simulink model "example"  (R2020b)
settings: Solver=ode45  StartTime=0.0  StopTime=10.0  RelTol=1e-3
InitFcn:
  | ac_testbed_setup
undefined symbols (not defined in the file): mpm, PD, QD, QG, VA, VM
libraries: SimMATPOWERbase x6, simulink x1
settings Model: Creator=hauswirth  LastModifiedBy=lukas
settings DataIOCC: SaveFormat=StructureWithTime  ReturnWorkspaceOutputs=off
settings OptimizationCC: LifeSpan=inf
settings DebuggingCC: SFExecutionAtInitializationDiag=none  ArithmeticOperatorsInVariantConditions=warning
settings HardwareCC: ProdBitPerSizeT=32  ProdBitPerPtrDiffT=32  ProdWordSize=32  ProdHWDeviceType=Specified
settings SFSimCC: CustomCodeUndefinedFunction=UseInterfaceOnly
settings CodeAppCC: StateflowObjectComments=on

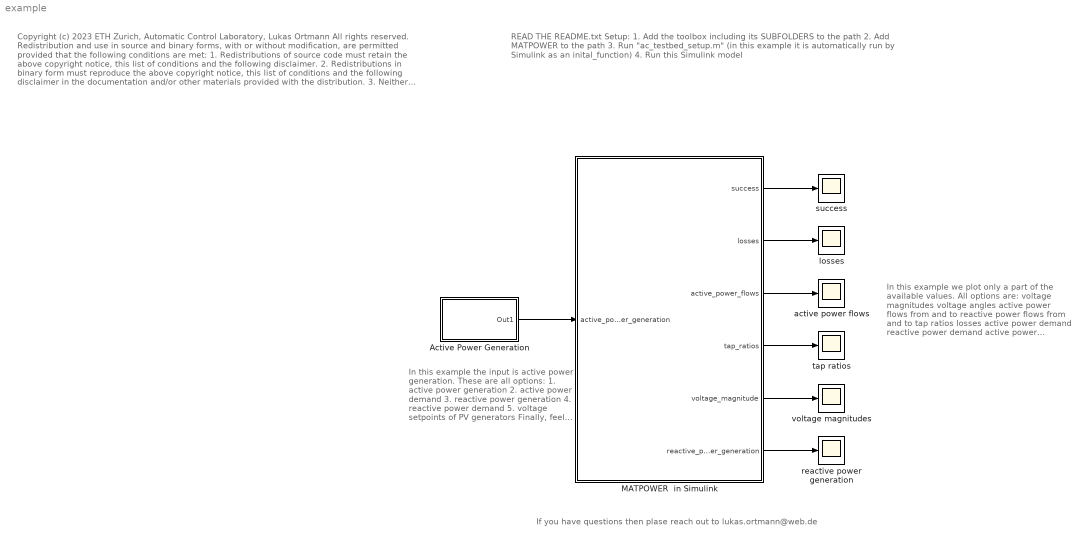
== system example ==
  note: Copyright (c) 2023 ETH Zurich, Automatic Control Laboratory, Lukas Ortmann
      | All rights reserved.
      |
      | Redistribution and use in source and binary forms, with or without
      | modification, are permitted provided that the following conditions are
      | met:
      |
      | 1. Redistributions of source code must retain the above copyright
      | notice, this list of conditions and the following disclaimer.
      |
      | 2. Redistributions in binary form must reproduce the above copyright
      | notice, this list of conditions and the following disclaimer in the
      | documentation and/or other materials provided with the distribution.
      |
      | 3. Neither the name of the copyright holder nor the names of its
      | contributors may be used to endorse or promote products derived from
      | this software without specific prior written permission.
      |
      | THIS SOFTWARE IS PROVIDED BY THE COPYRIGHT HOLDERS AND CONTRIBUTORS "AS
      | IS" AND ANY EXPRESS OR IMPLIED WARRANTIES, INCLUDING, BUT NOT LIMITED
      | TO, THE IMPLIED WARRANTIES OF MERCHANTABILITY AND FITNESS FOR A
      | PARTICULAR PURPOSE ARE DISCLAIMED. IN NO EVENT SHALL THE COPYRIGHT
      | HOLDER OR CONTRIBUTORS BE LIABLE FOR ANY DIRECT, INDIRECT, INCIDENTAL,
      | SPECIAL, EXEMPLARY, OR CONSEQUENTIAL DAMAGES (INCLUDING, BUT NOT LIMITED
      | TO, PROCUREMENT OF SUBSTITUTE GOODS OR SERVICES; LOSS OF USE, DATA, OR
      | PROFITS; OR BUSINESS INTERRUPTION) HOWEVER CAUSED AND ON ANY THEORY OF
      | LIABILITY, WHETHER IN CONTRACT, STRICT LIABILITY, OR TORT (INCLUDING
      | NEGLIGENCE OR OTHERWISE) ARISING IN ANY WAY OUT OF THE USE OF THIS
      | SOFTWARE, EVEN IF ADVISED OF THE POSSIBILITY OF SUCH DAMAGE.
  note: READ THE README.txt
      | Setup:
      | 1. Add the toolbox including its SUBFOLDERS to the path
      | 2. Add MATPOWER to the path
      | 3. Run "ac_testbed_setup.m" (in this example it is automatically run by Simulink as an inital_function)
      | 4. Run this Simulink model
  note: If you have questions then plase reach out to lukas.ortmann@web.de
  note: In this example the input is active power generation. These are all options:
      | 1. active power generation
      | 2. active power demand
      | 3. reactive power generation
      | 4. reactive power demand
      | 5. voltage setpoints of PV generators
      |
      | Finally, feel free to extend the code to include switches or tap changers
  note: In this example we plot only a part of the available values. All options are:
      | voltage magnitudes
      | voltage angles
      | active power flows from and to
      | reactive power flows from and to
      | tap ratios
      | losses
      | active power demand
      | reactive power demand
      | active power generation
      | reactive power generation
  Active Power Generation : Subsystem
  MATPOWER  in Simulink : Subsystem
  active power flows : Scope
  losses : Scope
  reactive power generation : Scope
  success : Scope
  tap ratios : Scope
  voltage magnitudes : Scope
  wires:
  MATPOWER  in Simulink/1(success) -> success/1
  MATPOWER  in Simulink/5(voltage_magnitude) -> voltage magnitudes/1
  MATPOWER  in Simulink/4(tap_ratios) -> tap ratios/1
  MATPOWER  in Simulink/2(losses) -> losses/1
  MATPOWER  in Simulink/3(active_power_flows) -> active power flows/1
  Active Power Generation/1(Out1) -> MATPOWER  in Simulink/1(active_power_generation)
  MATPOWER  in Simulink/6(reactive_power_generation) -> reactive power generation/1

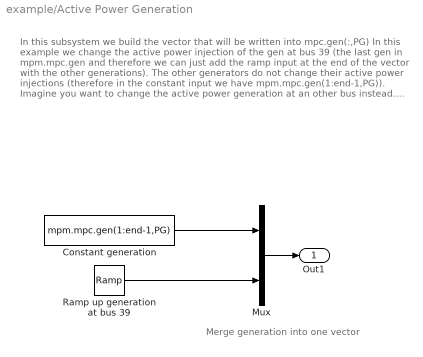
== system example/Active Power Generation ==
  note: Merge generation into one vector
  note: In this subsystem we build the vector that will be written into mpc.gen(:,PG)
      |
      | In this example we change the active power injection of the gen at bus 39 (the last gen in mpm.mpc.gen and therefore we can just add the ramp input at the end of the vector with the other generations).
      | The other generators do not change their active power injections (therefore in the constant input we have mpm.mpc.gen(1:end-1,PG)).
      |
      | Imagine you want to change the active power generation at an other bus instead. Overall, what you need to do is construct the vector that will be given to mpc.gen(:,PG). Therefore, find out the position in mpc.gen(:,PG) that corresponds to the generator you want to change. For example in the 39bus case of this example the generator at bus 30 is at position 1 of mpc.gen(:,PG).
      |
      | You can of course change all setpoints at the same time for all inputs you want
  Constant generation : Constant  Value=mpm.mpc.gen(1:end-1,PG)
  Mux : Mux  Inputs=2
  Ramp up generation at bus 39 : simulink/Sources/Ramp  slope=50  start=0  InitialOutput=1000
  Out1 : Outport
  wires:
  Mux/1 -> Out1/1
  Constant generation/1 -> Mux/1
  Ramp up generation at bus 39/1 -> Mux/2

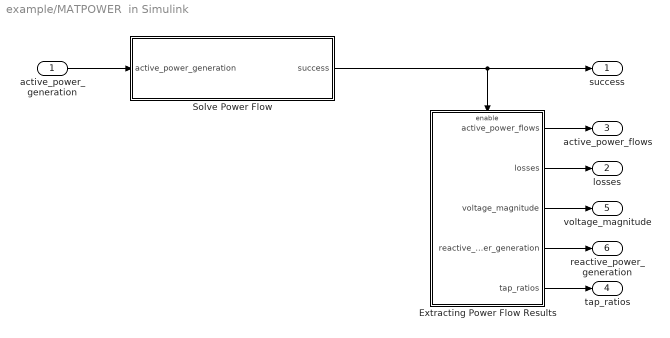
== system example/MATPOWER  in Simulink ==
  active_power_generation : Inport
  Extracting Power Flow Results : Subsystem
  Solve Power Flow : Subsystem
  success : Outport
  losses : Outport  Port=2
  active_power_flows : Outport  Port=3
  tap_ratios : Outport  Port=4
  voltage_magnitude : Outport  Port=5
  reactive_power_generation : Outport  Port=6
  wires:
  active_power_generation/1 -> Solve Power Flow/1(active_power_generation)
  Solve Power Flow/1(success) -> Extracting Power Flow Results/Enable, success/1
  Extracting Power Flow Results/1(active_power_flows) -> active_power_flows/1
  Extracting Power Flow Results/2(losses) -> losses/1
  Extracting Power Flow Results/5(tap_ratios) -> tap_ratios/1
  Extracting Power Flow Results/3(voltage_magnitude) -> voltage_magnitude/1
  Extracting Power Flow Results/4(reactive_power_generation) -> reactive_power_generation/1

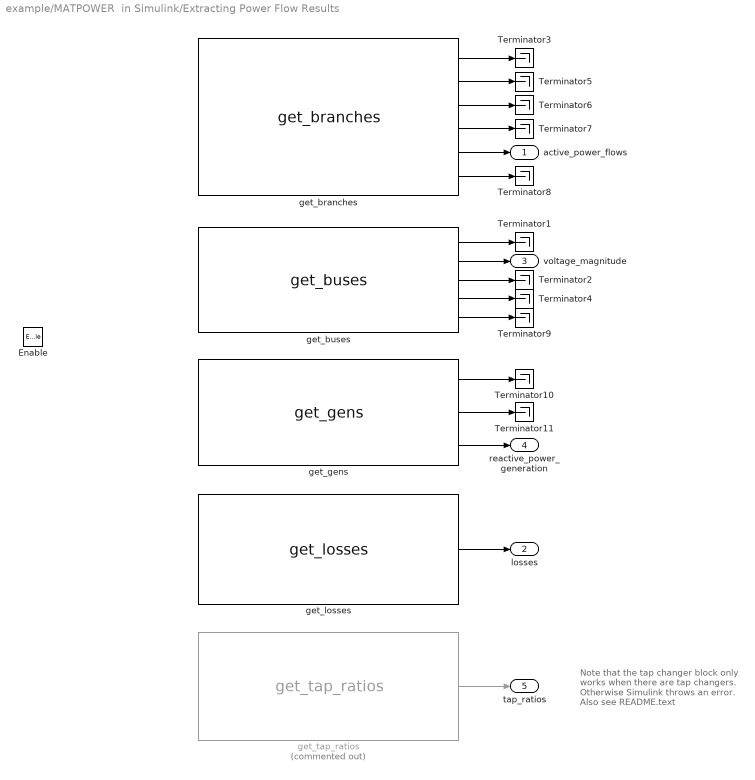
== system example/MATPOWER  in Simulink/Extracting Power Flow Results ==
  note: Note that the tap changer block only works when there are tap changers. Otherwise Simulink throws an error. Also see README.text
  Enable : EnablePort  PropagateVarSize=During execution
  Terminator{1..11} (11 alike) : Terminator
  get_branches : SimMATPOWERbase/get_branches  SystemSampleTime=1  VariantActivationTime=update diagram  Latency=0  AutoFrameSizeCalculation=off
  get_buses : SimMATPOWERbase/get_buses  SystemSampleTime=1  VariantActivationTime=update diagram  Latency=0  AutoFrameSizeCalculation=off
  get_gens : SimMATPOWERbase/get_gens  SystemSampleTime=1  VariantActivationTime=update diagram  Latency=0  AutoFrameSizeCalculation=off
  get_losses : SimMATPOWERbase/get_losses  SystemSampleTime=1  VariantActivationTime=update diagram  Latency=0  AutoFrameSizeCalculation=off
  get_tap_ratios : SimMATPOWERbase/get_tap_ratios  Commented=on  SystemSampleTime=1  VariantActivationTime=update diagram  Latency=0  AutoFrameSizeCalculation=off
  active_power_flows : Outport
  losses : Outport  Port=2
  voltage_magnitude : Outport  Port=3
  reactive_power_generation : Outport  Port=4
  tap_ratios : Outport  Port=5
  wires:
  get_gens/3 -> reactive_power_generation/1
  get_buses/5 -> Terminator9/1
  get_tap_ratios/1 -> tap_ratios/1
  get_gens/1 -> Terminator10/1
  get_buses/1 -> Terminator1/1
  get_buses/3 -> Terminator2/1
  get_buses/4 -> Terminator4/1
  get_branches/5 -> active_power_flows/1
  get_branches/2 -> Terminator5/1
  get_branches/4 -> Terminator7/1
  get_losses/1 -> losses/1
  get_branches/1 -> Terminator3/1
  get_buses/2 -> voltage_magnitude/1
  get_gens/2 -> Terminator11/1
  get_branches/6 -> Terminator8/1
  get_branches/3 -> Terminator6/1

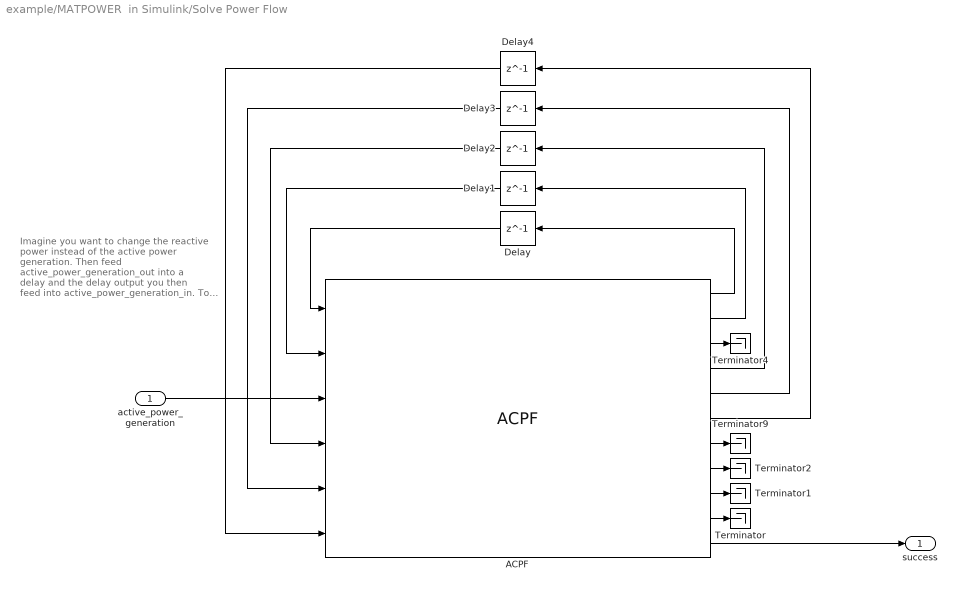
== system example/MATPOWER  in Simulink/Solve Power Flow ==
  note: Imagine you want to change the reactive power instead of the active power generation.
      | Then feed active_power_generation_out into a delay and the delay output you then feed into active_power_generation_in.
      | To change the reactive power do what we did here with the reactive power.
      |
      | You can of course change active and reactive power at the same time. Then just input whatever you want into reactive_power_generation_in and active_power_generation_in
  active_power_generation : Inport
  ACPF : SimMATPOWERbase/ACPF  SystemSampleTime=-1  VariantActivationTime=update diagram  Latency=0  AutoFrameSizeCalculation=off
  Delay : Delay  DelayLength=1  InitialCondition=mpm.mpc.bus(:,VM)
  Delay1 : Delay  DelayLength=1  InitialCondition=mpm.mpc.bus(:,VA)
  Delay2 : Delay  DelayLength=1  InitialCondition=mpm.mpc.gen(:,QG)
  Delay3 : Delay  DelayLength=1  InitialCondition=mpm.mpc.bus(:,PD)
  Delay4 : Delay  DelayLength=1  InitialCondition=mpm.mpc.bus(:,QD)
  Terminator{,1..2,4,9} (5 alike) : Terminator
  success : Outport
  wires:
  ACPF/7 -> Terminator9/1
  ACPF/10 -> Terminator/1
  ACPF/6 -> Delay4/1
  ACPF/11 -> success/1
  Delay4/1 -> ACPF/6
  ACPF/5 -> Delay3/1
  ACPF/9 -> Terminator1/1
  active_power_generation/1 -> ACPF/3
  Delay3/1 -> ACPF/5
  ACPF/8 -> Terminator2/1
  Delay2/1 -> ACPF/4
  Delay/1 -> ACPF/1
  ACPF/2 -> Delay1/1
  ACPF/1 -> Delay/1
  ACPF/4 -> Delay2/1
  ACPF/3 -> Terminator4/1
  Delay1/1 -> ACPF/2
